simulink model "PID"  (R2018b)
settings: Solver=FixedStepAuto  StartTime=0.0  StopTime=1  FixedStep=Ts  RelTol=1e-3
undefined symbols (not defined in the file): Gs, Gzz, K, Ka, Kd, Ki, Kp, L, Ts
libraries: simulink x1
settings Model: Creator=deepin  LastModifiedBy=deepin

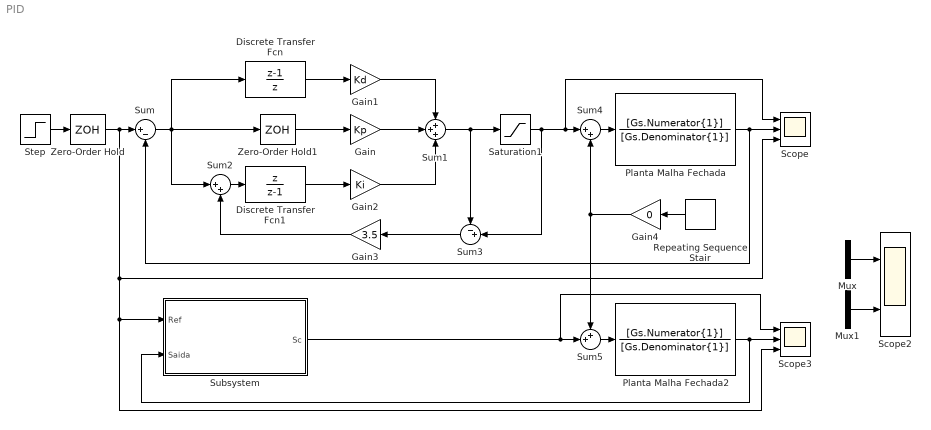
== system PID ==
  Discrete Transfer Fcn : DiscreteTransferFcn  Numerator=[1 -1]  Denominator=[1 0]  SampleTime=Ts
  Discrete Transfer Fcn1 : DiscreteTransferFcn  Numerator=[1 0]  Denominator=[1 -1]  SampleTime=Ts
  Gain : Gain  Gain=Kp
  Gain1 : Gain  Gain=Kd
  Gain2 : Gain  Gain=Ki
  Gain3 : Gain  Gain=3.5
  Gain4 : Gain  Gain=0
  Mux : Mux  Inputs=3
  Mux1 : Mux  Inputs=2
  Planta Malha Fechada : TransferFcn  Numerator=[Gs.Numerator{1}]  Denominator=[Gs.Denominator{1}]
  Planta Malha Fechada2 : TransferFcn  Numerator=[Gs.Numerator{1}]  Denominator=[Gs.Denominator{1}]
  Repeating Sequence Stair : simulink/Sources/Repeating Sequence Stair  OutValues=[0 1 0 -1].'  tsamp=Ts  OutMin=[]  OutMax=[]  OutDataTypeStr=double  OutputDataTypeScalingMode=double  OutDataType=fixdt(0,8)  ConRadixGroup=Best Precision: Vector-wise  OutScaling=2^-12
  Saturation1 : Saturate  UpperLimit=255  LowerLimit=-255
  Scope : Scope  NumInputPorts=3
  Scope2 : Scope  NumInputPorts=2
  Scope3 : Scope  NumInputPorts=3
  Step : Step  Time=Ts  After=1023  SampleTime=0
  Subsystem : Subsystem
  Sum : Sum  Inputs=|+-
  Sum1 : Sum  Inputs=+++
  Sum2 : Sum  Inputs=|++
  Sum3 : Sum  Inputs=-+|
  Sum4 : Sum  Inputs=|++
  Sum5 : Sum  Inputs=++|
  Zero-Order Hold : ZeroOrderHold  SampleTime=-1
  Zero-Order Hold1 : ZeroOrderHold  SampleTime=Ts
  wires:
  Sum/1 -> Sum2/1, Discrete Transfer Fcn/1, Zero-Order Hold1/1
  Discrete Transfer Fcn/1 -> Gain1/1
  Discrete Transfer Fcn1/1 -> Gain2/1
  Gain/1 -> Sum1/2
  Sum1/1 -> Sum3/1, Saturation1/1
  Gain1/1 -> Sum1/1
  Planta Malha Fechada/1 -> Sum/2, Scope/2
  Step/1 -> Zero-Order Hold/1
  Planta Malha Fechada2/1 -> Subsystem/2(Saida), Scope3/2
  Zero-Order Hold/1 -> Scope3/3, Subsystem/1(Ref), Scope/3, Sum/1
  Sum2/1 -> Discrete Transfer Fcn1/1
  Sum3/1 -> Gain3/1
  Gain3/1 -> Sum2/2
  Saturation1/1 -> Scope/1, Sum4/1, Sum3/2
  Sum4/1 -> Planta Malha Fechada/1
  Repeating Sequence Stair/1 -> Gain4/1
  Subsystem/1(Sc) -> Sum5/2, Scope3/1
  Sum5/1 -> Planta Malha Fechada2/1
  Gain4/1 -> Sum5/1, Sum4/2
  Zero-Order Hold1/1 -> Gain/1
  Gain2/1 -> Sum1/3
  Mux/1 -> Scope2/1
  Mux1/1 -> Scope2/2

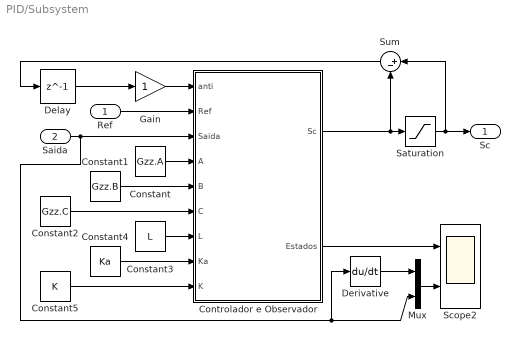
== system PID/Subsystem ==
  Ref : Inport
  Saida : Inport  Port=2
  Constant : Constant  Value=Gzz.A
  Constant1 : Constant  Value=Gzz.B
  Constant2 : Constant  Value=Gzz.C
  Constant3 : Constant  Value=L
  Constant4 : Constant  Value=Ka
  Constant5 : Constant  Value=K
  Controlador e Observador : MATLAB Function  TreatAsAtomicUnit=on  SystemSampleTime=Ts
  Delay : Delay  DelayLength=1  SampleTime=Ts
  Derivative : Derivative  CoefficientInTFapproximation=Ts
  Gain : Gain
  Mux : Mux  Inputs=2
  Saturation : Saturate  UpperLimit=255  LowerLimit=-255
  Scope2 : Scope  NumInputPorts=2
  Sum : Sum  Inputs=|+-
  Sc : Outport
  wires:
  Sum/1 -> Delay/1
  Controlador e Observador/1(Sc) -> Sum/2, Saturation/1
  Saida/1 -> Controlador e Observador/3(Saida), Mux/2, Derivative/1
  Saturation/1 -> Sc/1, Sum/1
  Controlador e Observador/2(Estados) -> Scope2/1
  Ref/1 -> Controlador e Observador/2(Ref)
  Constant/1 -> Controlador e Observador/4(A)
  Constant1/1 -> Controlador e Observador/5(B)
  Constant3/1 -> Controlador e Observador/7(L)
  Constant2/1 -> Controlador e Observador/6(C)
  Constant4/1 -> Controlador e Observador/8(Ka)
  Constant5/1 -> Controlador e Observador/9(K)
  Gain/1 -> Controlador e Observador/1(anti)
  Derivative/1 -> Mux/1
  Mux/1 -> Scope2/2
  Delay/1 -> Gain/1

== matlab function PID/Subsystem/Controlador e Observador ==
  data: anti input; Ref input; Saida input; Sc output; Estados output; A input; B input; C input; L input; Ka input; K input
function [Sc,Estados] = fcn(anti, Ref,Saida,A,B,C,L,Ka,K)

persistent EstadosA;
persistent ScA;
persistent int;
if isempty(EstadosA)
    EstadosA = [0; 0];
end
if isempty(ScA)
    ScA = 0;
end
if isempty(int)
    int = 0; 
end

%% Observador

EstadosA = A*EstadosA + B*ScA + L*(Saida-C'*EstadosA);

%% Controlador

int = int + Ref - Saida + anti; %Integrador
Sc  = 0;
Sc  = int*(-Ka) - K'*EstadosA; %Sinal de controle
ScA=Sc;
Int=int;
Estados=EstadosA;
